simulink model "mcb_bldc_sixstep_f28069mLaunchPad_r2020a"  (R2020a)
settings: Solver=FixedStepDiscrete  StartTime=0.0  StopTime=2  RelTol=1e-3  EnableMultiTasking=on
InitFcn:
  | mcb_bldc_sixstep_f28069mLaunchPad_data;
undefined symbols (not defined in the file): bldc, Down, GPTRIP1SEL, GPTRIP2SEL, inverter, PI_params, PWM_frequency, target, Ts, Ts_motor, Ts_motor_simscape, Ts_simulink, Ts_speed, TZ1, TZ2, Up
libraries: nesl_utility x14, fl_lib x9, mcbcontrolslib x8, simulink x8, c2802xlib x7, mcbpositiondecoderlib x5, c2806xlib x5, c280xlib x5, ee_lib x5, svdschedulerlib x2
(part 1 of 3)
settings Model: SILPILModeSetting=veronly  SILPILSystemUnderTest=refmodels  ExtModeTrigDuration=8  OrderedModelArguments=off  Creator=The MathWorks, Inc.  LastModifiedBy=Tefilus
settings SolverCC: AutoInsertRateTranBlk=on
settings DataIOCC: LimitDataPoints=on  SaveFormat=Array  SaveOutput=off  SaveTime=off  ReturnWorkspaceOutputs=off
settings OptimizationCC: DefaultParameterBehavior=Inlined  DefaultUnderspecifiedDataType=single  OptimizeBlockIOStorage=off  BufferReuse=off  GlobalBufferReuse=off  ExpressionFolding=off  ExpressionDepthLimit=2147483647  LocalBlockOutputs=off  InitFltsAndDblsToZero=on  NoFixptDivByZeroProtection=on  EfficientFloat2IntCast=on  EfficientMapNaN2IntZero=off  LifeSpan=inf  MaxStackSize=1024  OptimizeDataStoreBuffers=off  BusAssignmentInplaceUpdate=off  DenormalBehavior=FlushToZero  EfficientTunableParamExpr=on
settings DebuggingCC: AlgebraicLoopMsg=error  ArtificialAlgebraicLoopMsg=error  CheckSSInitialOutputMsg=off  MergeDetectMultiDrivingBlocksExec=none  SolverPrmCheckMsg=warning  InheritedTsInSrcMsg=none  MultiTaskDSMMsg=none  MultiTaskCondExecSysMsg=none  TasksWithSamePriorityMsg=none  SigSpecEnsureSampleTimeMsg=none  ParameterPrecisionLossMsg=none  ParameterTunabilityLossMsg=error  FcnCallInpInsideContextMsg=warning  AllowSymbolicDim=off  StateNameClashWarn=warning  SFUnexpectedBacktrackingDiag=warning  SFNoUnconditionalDefaultTransitionDiag=warning  SFExecutionAtInitializationDiag=none  ArithmeticOperatorsInVariantConditions=warning
settings HardwareCC: ProdBitPerChar=16  ProdBitPerInt=16  ProdBitPerPointer=32  ProdBitPerSizeT=32  ProdBitPerPtrDiffT=32  ProdLargestAtomicInteger=Integer  ProdLargestAtomicFloat=None  ProdWordSize=16  ProdLongLongMode=on  ProdHWDeviceType=Texas Instruments->C2000  TargetBitPerChar=16  TargetBitPerInt=16  TargetLargestAtomicInteger=Integer  TargetLongLongMode=on  TargetIntDivRoundTo=Zero  TargetEndianess=LittleEndian  TargetWordSize=16  TargetHWDeviceType=Texas Instruments->C2000  ProdEqTarget=off
settings ModelReferenceCC: PropagateSignalLabelsOutOfModel=off
settings SFSimCC: SimUseLocalCustomCode=off  MATLABDynamicMemAlloc=off
settings RTWCC: SystemTargetFile=ert.tlc  HardwareBoard=TI Piccolo F28069M LaunchPad  TLCOptions=-aInlineSetEventsForThisBaseRateFcn=TLC_FALSE -aSuppressMultiTaskScheduler=TLC_FALSE -aRateBasedStepFcn=1  TemplateMakefile=ert_default_tmf  PostCodeGenCommand=; codertarget.postCodeGenHookCommand(h)  GenerateReport=on  RTWUseLocalCustomCode=off  Toolchain=Texas Instruments Code Composer Studio (C2000)  IncludeHyperlinkInReport=on  GenerateTraceInfo=on  GenerateTraceReport=on  GenerateTraceReportSl=on  GenerateTraceReportSf=on  GenerateTraceReportEml=on
settings CodeAppCC: IgnoreCustomStorageClasses=off  CustomSymbolStrType=$N$R$M  StateflowObjectComments=on  InternalIdentifier=Classic
settings ERTTargetCC: TargetFcnLib=ansi_tfl_tmw_new.mat  CodeReplacementLibrary=TI C28x  MultiwordLength=2048  ParMdlRefBuildCompliant=off  CompOptLevelCompliant=off  ConcurrentExecutionCompliant=off  CPPClassGenCompliant=off  ExtModeStaticAllocSize=2000  ExtModeMexFile=TIC2000ExternalModeOpen  ExtModeIntrfLevel=Level2 - Open  ConvertIfToSwitch=off  SuppressUnreachableDefaultCases=off  MemSecPackage=tic2000demospkg
settings ConfigComp: CovMetricSettings=dw  CovSaveCumulativeToWorkspaceVar=on  CovSaveSingleToWorkspaceVar=on  CovExternalEMLEnable=off  CovSFcnEnable=off

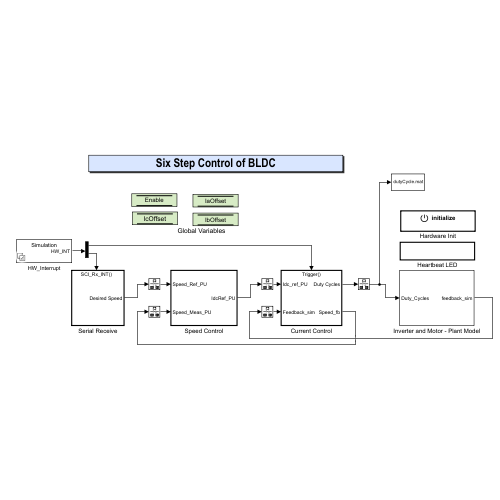
[thumbnail: Simulink's stored preview of the top-level diagram]
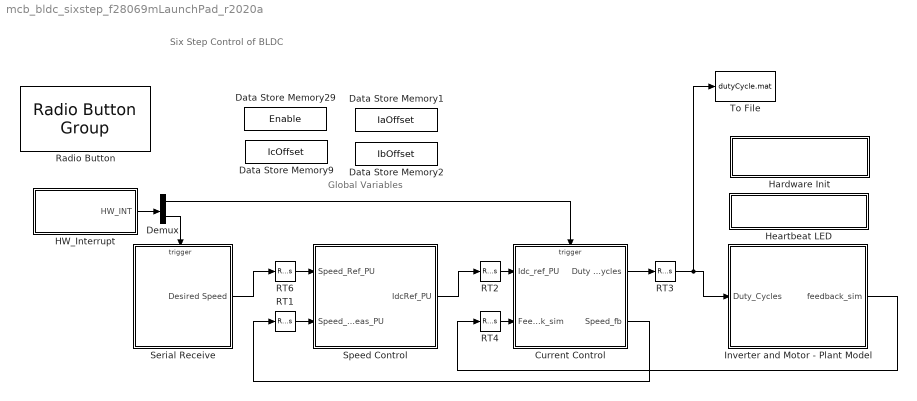
== system mcb_bldc_sixstep_f28069mLaunchPad_r2020a ==
  note: Six Step Control of BLDC
  note: Global Variables
  Current Control : Subsystem
      settings: RTWSystemCode=Nonreusable function
  Data Store Memory1 : DataStoreMemory  DataStoreName=IaOffset  InitialValue=inverter.CtSensAOffset  ShowAdditionalParam=off
  Data Store Memory2 : DataStoreMemory  DataStoreName=IbOffset  InitialValue=inverter.CtSensBOffset  ShowAdditionalParam=off
  Data Store Memory29 : DataStoreMemory  DataStoreName=Enable  ShowAdditionalParam=off  OutDataTypeStr=boolean
  Data Store Memory9 : DataStoreMemory  DataStoreName=IcOffset  InitialValue=inverter.CtSensBOffset  ShowAdditionalParam=off
  Demux : Demux  Outputs=2
  HW_Interrupt : Subsystem  Variant=on  VariantControlMode=Expression
  Hardware Init : Subsystem  TreatAsAtomicUnit=on
  Heartbeat LED : Subsystem  TreatAsAtomicUnit=on
  Inverter and Motor - Plant Model : Subsystem
  RT1 : RateTransition  Deterministic=off  OutPortSampleTime=Ts_speed
  RT{2..4,6} (4 alike) : RateTransition  Deterministic=off
  Radio Button : RadioButtonGroup  LabelPosition=Hide  SelectedLabel=Quadrature Encoder  ButtonGroupName=Speed_Feedback
      settings: Values={{'Quadrature Encoder', 'Hall'}, [0 1]}
  Serial Receive : Subsystem  SystemSampleTime=1e-3
  Speed Control : Subsystem  TreatAsAtomicUnit=on  SystemSampleTime=Ts_speed
  To File : ToFile  Filename=dutyCycle.mat  SaveFormat=Timeseries
  wires:
  RT3/1 -> To File/1, Inverter and Motor - Plant Model/1(Duty_Cycles)
  Inverter and Motor - Plant Model/1(feedback_sim) -> RT4/1
  Demux/1 -> Current Control/Trigger
  RT6/1 -> Speed Control/1(Speed_Ref_PU)
  RT1/1 -> Speed Control/2(Speed_Meas_PU)
  Speed Control/1(IdcRef_PU) -> RT2/1
  Demux/2 -> Serial Receive/Trigger
  Current Control/1(Duty Cycles) -> RT3/1
  HW_Interrupt/1(HW_INT) -> Demux/1
  Current Control/2(Speed_fb) -> RT1/1
  RT4/1 -> Current Control/2(Feedback_sim)
  Serial Receive/1(Desired Speed) -> RT6/1
  RT2/1 -> Current Control/1(Idc_ref_PU)

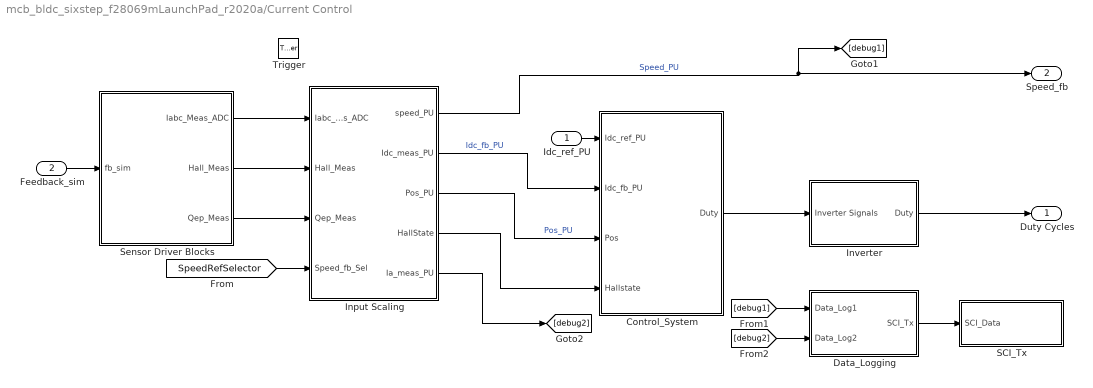
== system mcb_bldc_sixstep_f28069mLaunchPad_r2020a/Current Control ==
  Idc_ref_PU : Inport
  Feedback_sim : Inport  Port=2
  Trigger : TriggerPort  TriggerType=function-call  VariantControl=Variant  PortDimensions=1
  Control_System : Subsystem
  Data_Logging : Subsystem
  Input Scaling : Subsystem
  Inverter : Subsystem  Variant=on  VariantControlMode=Expression
  SCI_Tx : Subsystem  Variant=on  VariantControlMode=Expression
  Sensor Driver Blocks : Subsystem  Variant=on  VariantControlMode=Expression
  Duty Cycles : Outport  InitialOutput=0  VectorParamsAs1DForOutWhenUnconnected=off
  Speed_fb : Outport  Port=2  InitialOutput=0  VectorParamsAs1DForOutWhenUnconnected=off
  wires:
  [debug1] -> Data_Logging/1(Data_Log1)
  [debug2] -> Data_Logging/2(Data_Log2)
  Inverter/1(Duty) -> Duty Cycles/1
  Data_Logging/1(SCI_Tx) -> SCI_Tx/1(SCI_Data)
  [SpeedRefSelector] -> Input Scaling/4(Speed_fb_Sel)
  Sensor Driver Blocks/1(Iabc_Meas_ADC) -> Input Scaling/1(Iabc_meas_ADC)
  Feedback_sim/1 -> Sensor Driver Blocks/1(fb_sim)
  Idc_ref_PU/1 -> Control_System/1(Idc_ref_PU)
  Input Scaling/2(Idc_meas_PU) -> Control_System/2(Idc_fb_PU)  "Idc_fb_PU"
  Input Scaling/3(Pos_PU) -> Control_System/3(Pos)  "Pos_PU"
  Input Scaling/4(HallState) -> Control_System/4(Hallstate)
  Input Scaling/1(speed_PU) -> [debug1], Speed_fb/1  "Speed_PU"
  Input Scaling/5(Ia_meas_PU) -> [debug2]
  Sensor Driver Blocks/2(Hall_Meas) -> Input Scaling/2(Hall_Meas)
  Sensor Driver Blocks/3(Qep_Meas) -> Input Scaling/3(Qep_Meas)
  Control_System/1(Duty) -> Inverter/1(Inverter Signals)

== system mcb_bldc_sixstep_f28069mLaunchPad_r2020a/HW_Interrupt ==
  Code generation : Subsystem  VariantControl=(codegen)
  Simulation : Subsystem  VariantControl=(sim)
  HW_INT : Outport

== system mcb_bldc_sixstep_f28069mLaunchPad_r2020a/Hardware Init ==
  6PWM_Mode : Constant  Priority=1000  Value=0x3A16  OutDataTypeStr=uint16  SampleTime=-1
  ADC_Gain_Setting : Constant  Priority=1000  Value=inverter.SPI_Gain_Setting  OutDataTypeStr=uint16  SampleTime=-1
  Event Listener : EventListener  DisableCoverage=on  EventName=reset
  Mux : Mux  Inputs=2
  Variant Subsystem : Subsystem  Variant=on  VariantControlMode=Expression
  wires:
  6PWM_Mode/1 -> Mux/1
  ADC_Gain_Setting/1 -> Mux/2
  Mux/1 -> Variant Subsystem/1(In1)

== system mcb_bldc_sixstep_f28069mLaunchPad_r2020a/Heartbeat LED ==
  note: Heartbeat LED 1HZ
  Heartbeat LED : Subsystem  Variant=on  VariantControlMode=Expression
  RED_LED : Constant  OutDataTypeStr=uint16  SampleTime=0.5
  wires:
  RED_LED/1 -> Heartbeat LED/1(In1)

== system mcb_bldc_sixstep_f28069mLaunchPad_r2020a/Inverter and Motor - Plant Model ==
  Duty_Cycles : Inport
  Codegeneration : Subsystem
  Simulation : Subsystem
  Variant Sink : VariantSink  VariantControlMode=Expression
  Variant Source : VariantSource  VariantControlMode=Expression
  feedback_sim : Outport  VectorParamsAs1DForOutWhenUnconnected=off
  wires:
  Codegeneration/1(fb_codegen) -> Variant Source/1
  Variant Sink/1 -> Codegeneration/1(Duty_Cycles)
  Variant Source/1 -> feedback_sim/1
  Duty_Cycles/1 -> Variant Sink/1
  Variant Sink/2 -> Simulation/1(Duty_Cycles)
  Simulation/1(fb_sim) -> Variant Source/2

== system mcb_bldc_sixstep_f28069mLaunchPad_r2020a/Serial Receive ==
  SCI_Rx_INT : TriggerPort  TriggerType=function-call  VariantControl=Variant
  Data Store Write : DataStoreWrite  DataStoreName=Enable
  Data Type Conversion1 : DataTypeConversion  OutDataTypeStr=dataType  RndMeth=Simplest
  Data Type Conversion3 : DataTypeConversion  OutDataTypeStr=boolean  RndMeth=Simplest
  Data_Conditioning : Subsystem
  Demux : Demux  Outputs=2
  SCI_Rx : Subsystem  Variant=on  VariantControlMode=Expression
  Desired Speed : Outport  VectorParamsAs1DForOutWhenUnconnected=off
  wires:
  SCI_Rx/1(Data) -> Data_Conditioning/1(In1)
  Data Type Conversion1/1 -> Desired Speed/1
  Demux/2 -> Data Type Conversion3/1
  Data_Conditioning/1(Out1) -> Demux/1
  Demux/1 -> Data Type Conversion1/1
  Data Type Conversion3/1 -> Data Store Write/1

== system mcb_bldc_sixstep_f28069mLaunchPad_r2020a/Speed Control ==
  Speed_Ref_PU : Inport
  Speed_Meas_PU : Inport  Port=2
  PI_Controller_Speed : Subsystem
  Scope : Scope  NumInputPorts=2
  Speed_Ref_Selector : Subsystem
  IdcRef_PU : Outport  VectorParamsAs1DForOutWhenUnconnected=off
  wires:
  PI_Controller_Speed/1(Idc_ref) -> IdcRef_PU/1
  Speed_Meas_PU/1 -> Scope/2, PI_Controller_Speed/2(N_fb), Speed_Ref_Selector/2(Speed_Ref_Open)  "Speed_fb"
  Speed_Ref_PU/1 -> Speed_Ref_Selector/1(Speed_Ref_In)  "SpeedRef"
  Speed_Ref_Selector/1(Speed_Ref_PU) -> Scope/1, PI_Controller_Speed/1(N_ref)  "Speed_Ref"

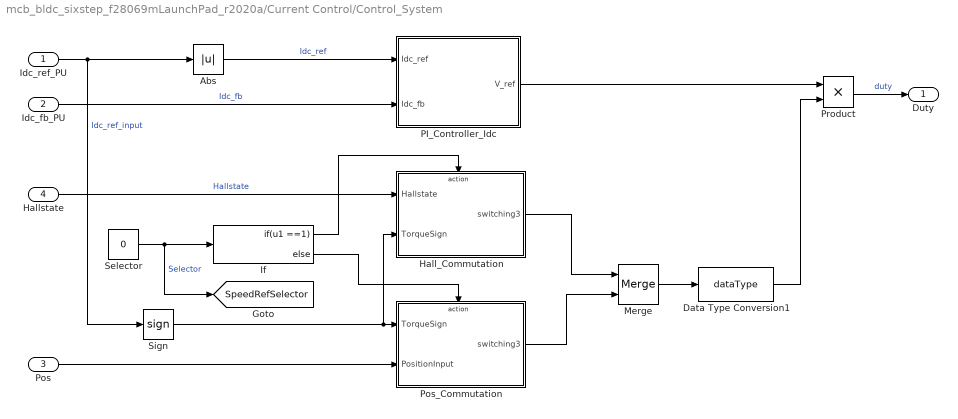
== system mcb_bldc_sixstep_f28069mLaunchPad_r2020a/Current Control/Control_System ==
  Idc_ref_PU : Inport
  Idc_fb_PU : Inport  Port=2
  Pos : Inport  Port=3
  Hallstate : Inport  Port=4
  Abs : Abs
  Data Type Conversion1 : DataTypeConversion  OutDataTypeStr=dataType  RndMeth=Simplest
  Hall_Commutation : Subsystem
  If : If  IfExpression=u1 ==1
  Merge : Merge
  PI_Controller_Idc : Subsystem
  Pos_Commutation : Subsystem
  Product : Product  RndMeth=Simplest  OutDataTypeStr=Inherit: Same as first input
  Selector : Constant  Value=0  OutDataTypeStr=uint16  SampleTime=-1
  Sign : Signum
  Duty : Outport  VectorParamsAs1DForOutWhenUnconnected=off
  tag scope: SpeedRefSelector=global
  wires:
  Hallstate/1 -> Hall_Commutation/1(Hallstate)  "Hallstate"
  Pos/1 -> Pos_Commutation/2(PositionInput)
  If/1 -> Hall_Commutation/Action
  If/2 -> Pos_Commutation/Action
  Pos_Commutation/1(switching3) -> Merge/2
  Hall_Commutation/1(switching3) -> Merge/1
  Merge/1 -> Data Type Conversion1/1
  Idc_fb_PU/1 -> PI_Controller_Idc/2(Idc_fb)  "Idc_fb"
  Abs/1 -> PI_Controller_Idc/1(Idc_ref)  "Idc_ref"
  PI_Controller_Idc/1(V_ref) -> Product/1
  Idc_ref_PU/1 -> Sign/1, Abs/1  "Idc_ref_input"
  Product/1 -> Duty/1  "duty"
  Selector/1 -> [SpeedRefSelector], If/1  "Selector"
  Sign/1 -> Hall_Commutation/2(TorqueSign), Pos_Commutation/1(TorqueSign)
  Data Type Conversion1/1 -> Product/2

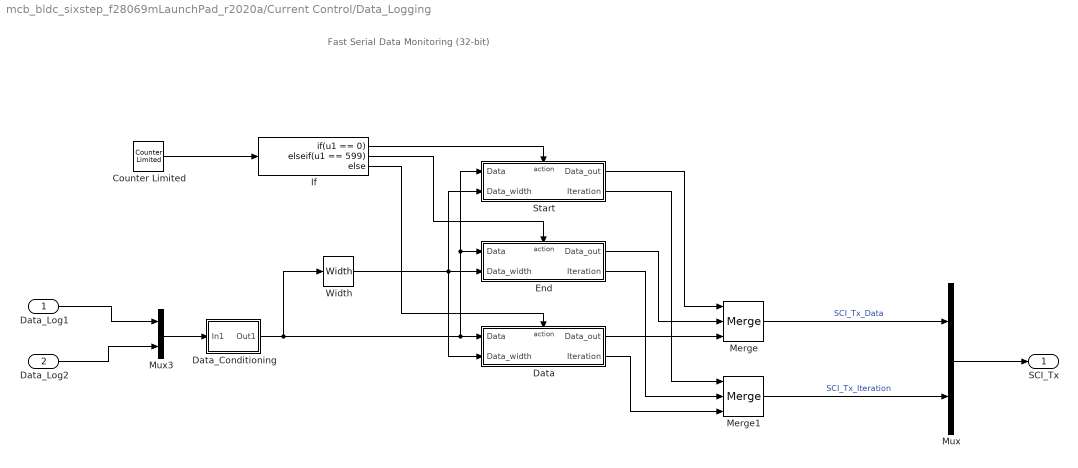
== system mcb_bldc_sixstep_f28069mLaunchPad_r2020a/Current Control/Data_Logging ==
  note: Fast Serial Data Monitoring (32-bit)
  Data_Log1 : Inport
  Data_Log2 : Inport  Port=2
  Counter Limited : simulink/Sources/Counter Limited  uplimit=599  tsamp=-1
  Data : Subsystem  TreatAsAtomicUnit=on
  Data_Conditioning : Subsystem
  End : Subsystem  TreatAsAtomicUnit=on
  If : If  IfExpression=u1 == 0  ElseIfExpressions=u1 == 599
  Merge : Merge  Inputs=3
  Merge1 : Merge  Inputs=3
  Mux : Mux  Inputs=2
  Mux3 : Mux  Inputs=2
  Start : Subsystem  TreatAsAtomicUnit=on
  Width : Width  OutDataTypeMode=All ports same datatype  DataType=uint16
  SCI_Tx : Outport
  wires:
  If/3 -> Data/Action
  Data/1(Data_out) -> Merge/3
  Width/1 -> Data/2(Data_width), Start/2(Data_width), End/2(Data_width)
  Merge/1 -> Mux/1  "SCI_Tx_Data"
  Counter Limited/1 -> If/1
  Start/2(Iteration) -> Merge1/1
  Start/1(Data_out) -> Merge/1
  If/2 -> End/Action
  Merge1/1 -> Mux/2  "SCI_Tx_Iteration"
  If/1 -> Start/Action
  End/1(Data_out) -> Merge/2
  End/2(Iteration) -> Merge1/2
  Data/2(Iteration) -> Merge1/3
  Data_Log1/1 -> Mux3/1
  Data_Conditioning/1(Out1) -> Width/1, Start/1(Data), End/1(Data), Data/1(Data)
  Mux/1 -> SCI_Tx/1
  Mux3/1 -> Data_Conditioning/1(In1)
  Data_Log2/1 -> Mux3/2

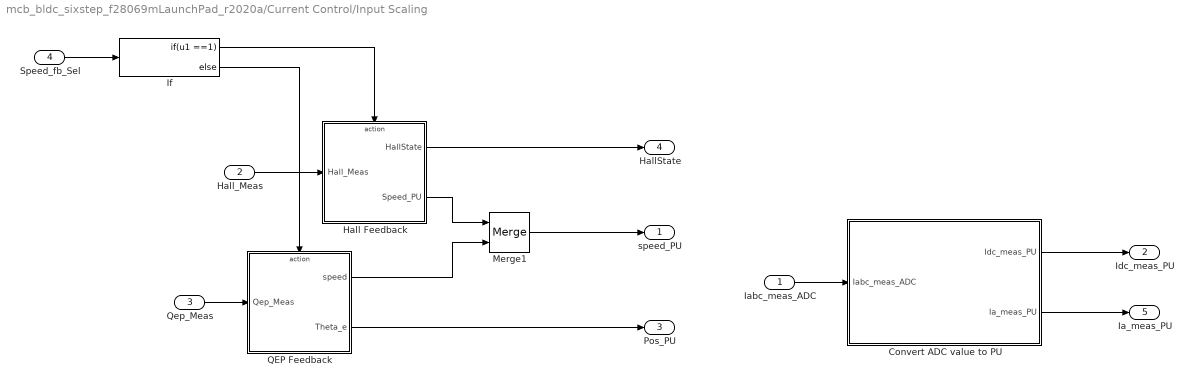
== system mcb_bldc_sixstep_f28069mLaunchPad_r2020a/Current Control/Input Scaling ==
  Iabc_meas_ADC : Inport
  Hall_Meas : Inport  Port=2
  Qep_Meas : Inport  Port=3
  Speed_fb_Sel : Inport  Port=4
  Convert ADC value to PU : Subsystem
  Hall Feedback : Subsystem  TreatAsAtomicUnit=on
  If : If  IfExpression=u1 ==1
  Merge1 : Merge
  QEP Feedback : Subsystem  TreatAsAtomicUnit=on
  speed_PU : Outport  InitialOutput=0  VectorParamsAs1DForOutWhenUnconnected=off
  Idc_meas_PU : Outport  Port=2  VectorParamsAs1DForOutWhenUnconnected=off
  Pos_PU : Outport  Port=3  InitialOutput=0  VectorParamsAs1DForOutWhenUnconnected=off
  HallState : Outport  Port=4  InitialOutput=0  VectorParamsAs1DForOutWhenUnconnected=off
  Ia_meas_PU : Outport  Port=5  VectorParamsAs1DForOutWhenUnconnected=off
  wires:
  If/2 -> QEP Feedback/Action
  Convert ADC value to PU/2(Ia_meas_PU) -> Ia_meas_PU/1
  Convert ADC value to PU/1(Idc_meas_PU) -> Idc_meas_PU/1
  QEP Feedback/1(speed) -> Merge1/2
  Hall Feedback/2(Speed_PU) -> Merge1/1
  Iabc_meas_ADC/1 -> Convert ADC value to PU/1(Iabc_meas_ADC)
  QEP Feedback/2(Theta_e) -> Pos_PU/1
  Merge1/1 -> speed_PU/1
  Speed_fb_Sel/1 -> If/1
  Hall_Meas/1 -> Hall Feedback/1(Hall_Meas)
  Qep_Meas/1 -> QEP Feedback/1(Qep_Meas)
  If/1 -> Hall Feedback/Action
  Hall Feedback/1(HallState) -> HallState/1

== system mcb_bldc_sixstep_f28069mLaunchPad_r2020a/Current Control/Inverter ==
  Inverter Signals : Inport
  " Code Generation" : Subsystem  VariantControl=(codegen)
  Simulation : Subsystem  VariantControl=(sim)
  Duty : Outport  VectorParamsAs1DForOutWhenUnconnected=off

== system mcb_bldc_sixstep_f28069mLaunchPad_r2020a/Current Control/SCI_Tx ==
  SCI_Data : Inport
  " Code Generation" : Subsystem  VariantControl=(codegen)
  Simulation : Subsystem  VariantControl=(sim)

== system mcb_bldc_sixstep_f28069mLaunchPad_r2020a/Current Control/Sensor Driver Blocks ==
  fb_sim : Inport
  Sensor Driver Blocks (codegen) : Subsystem  VariantControl=(codegen)
  Sensor Driver Blocks (sim) : Subsystem  VariantControl=(sim)
  Iabc_Meas_ADC : Outport
  Hall_Meas : Outport  Port=2
  Qep_Meas : Outport  Port=3

== system mcb_bldc_sixstep_f28069mLaunchPad_r2020a/HW_Interrupt/Code generation ==
  HWI_ADCINT1 : svdschedulerlib/Hardware Interrupt v2  ISRGroup=ADC - Analog to Digital Converter  ISRName=ADCA1_INT  ISRNumber=32  NumEventsToServe=1  EventsList={'on','EOC event','1';'off','Overflow event','2';'off','Custom event','3'}  SelectedEvents={'event1'}  TaskPriority=30  DisablePreemption=off  ClearInterruptFlagsAtEndOfEvent=on  InterruptDefinitionFile=$(TARGET_ROOT)/registry/interrupts/F2837xS_interrupts.xml  HardwareBoard=F2837x  EnableSimPort=off
  HWI_SCIRXINTA : svdschedulerlib/Hardware Interrupt v2  ISRGroup=ADC - Analog to Digital Converter  ISRName=ADCA1_INT  ISRNumber=32  NumEventsToServe=1  EventsList={'on','EOC event','1';'off','Overflow event','2';'off','Custom event','3'}  SelectedEvents={'event1'}  TaskPriority=50  DisablePreemption=on  ClearInterruptFlagsAtEndOfEvent=on  InterruptDefinitionFile=$(TARGET_ROOT)/registry/interrupts/F2837xS_interrupts.xml  HardwareBoard=F2837x  EnableSimPort=off
  Mux : Mux  Inputs=2
  HW_INT : Outport
  wires:
  HWI_SCIRXINTA/1 -> Mux/2
  HWI_ADCINT1/1 -> Mux/1
  Mux/1 -> HW_INT/1

== system mcb_bldc_sixstep_f28069mLaunchPad_r2020a/HW_Interrupt/Simulation ==
  ADCINT1 : simulink/Ports & Subsystems/Function-Call Generator  sample_time=Ts  numberOfIterations=1  DisallowWideOutput=off
  Mux : Mux  Inputs=2
  SCI_Rx_INT : simulink/Ports & Subsystems/Function-Call Generator  sample_time=0.1  numberOfIterations=1  DisallowWideOutput=off
  HW_INT : Outport
  wires:
  SCI_Rx_INT/1 -> Mux/2
  ADCINT1/1 -> Mux/1
  Mux/1 -> HW_INT/1

== system mcb_bldc_sixstep_f28069mLaunchPad_r2020a/Hardware Init/Variant Subsystem ==
  In1 : Inport
  Code Generation : Subsystem  VariantControl=(codegen)
  Simulation : Subsystem  VariantControl=(sim)

== system mcb_bldc_sixstep_f28069mLaunchPad_r2020a/Heartbeat LED/Heartbeat LED ==
  In1 : Inport
  Code generation : Subsystem  VariantControl=(codegen)
  Simulation : Subsystem  VariantControl=(sim)

== system mcb_bldc_sixstep_f28069mLaunchPad_r2020a/Inverter and Motor - Plant Model/Codegeneration ==
  Duty_Cycles : Inport
  Bus Creator : BusCreator  Inputs=3
  Ground : Ground
  Terminator : Terminator
  fb_codegen : Outport  VectorParamsAs1DForOutWhenUnconnected=off
  wires:
  Duty_Cycles/1 -> Terminator/1
  Bus Creator/1 -> fb_codegen/1
  Ground/1 -> Bus Creator/3, Bus Creator/2, Bus Creator/1

== system mcb_bldc_sixstep_f28069mLaunchPad_r2020a/Inverter and Motor - Plant Model/Simulation ==
  Duty_Cycles : Inport
  Bus Creator : BusCreator  Inputs=3
  Inverter and Motor : Subsystem  VariantControl=get_param([bdroot '/Plant'],'Value')=='0'
  Load_Profile (Torque) : Subsystem
  RT1 : RateTransition  Deterministic=off  OutPortSampleTime=Ts_simulink
  RT2 : RateTransition  Deterministic=off  OutPortSampleTime=Ts_simulink
  RT3 : RateTransition  Deterministic=off  OutPortSampleTime=Ts_simulink
  Sensor_Measurements : Subsystem
  fb_sim : Outport
  wires:
  RT2/1 -> Sensor_Measurements/3(Hall)
  Sensor_Measurements/2(Pos_mech) -> Bus Creator/2  "Pos_fb"
  RT1/1 -> Sensor_Measurements/2(Pos)
  Bus Creator/1 -> fb_sim/1
  Sensor_Measurements/1(Iabc meas ADC) -> Bus Creator/1  "Iabc_fb"
  Sensor_Measurements/3(HallState) -> Bus Creator/3  "Hall_fb"
  Duty_Cycles/1 -> Inverter and Motor/1(Duty_Cycles)
  Load_Profile (Torque)/1(Load_Trq) -> Inverter and Motor/2(Load)
  Inverter and Motor/1(Iabc) -> RT3/1
  Inverter and Motor/2(Theta) -> RT1/1
  Inverter and Motor/3(Hall) -> RT2/1
  RT3/1 -> Sensor_Measurements/1(Iabc meas)

== system mcb_bldc_sixstep_f28069mLaunchPad_r2020a/Serial Receive/Data_Conditioning ==
  In1 : Inport
  Data Type Conversion1 : DataTypeConversion  OutDataTypeStr=single  RndMeth=Simplest
  Data Type Conversion2 : DataTypeConversion  OutDataTypeStr=fixdt(1,16,12)  ConvertRealWorld=Stored Integer (SI)  RndMeth=Simplest
  Out1 : Outport  VectorParamsAs1DForOutWhenUnconnected=off
  wires:
  Data Type Conversion1/1 -> Out1/1
  In1/1 -> Data Type Conversion2/1
  Data Type Conversion2/1 -> Data Type Conversion1/1

== system mcb_bldc_sixstep_f28069mLaunchPad_r2020a/Serial Receive/SCI_Rx ==
  Code Generation : Subsystem  VariantControl=(codegen)
  Simulation : Subsystem  VariantControl=(sim)
  Data : Outport

== system mcb_bldc_sixstep_f28069mLaunchPad_r2020a/Speed Control/PI_Controller_Speed ==
  N_ref : Inport
  N_fb : Inport  Port=2
  Data Store Read2 : DataStoreRead  DataStoreName=Enable
  Discrete PI Controller with anti-windup & reset : mcbcontrolslib/Discrete PI Controller  with anti-windup & reset  Controller=PI  UpperSaturationLimit=1  LowerSaturationLimit=-1  IntegratorRTWStateStorageClass=Auto  FilterRTWStateStorageClass=Auto  ParallelPVariant=ExternalParameters  IdealPVariant=Disabled  IVariant=ExternalParameters  DVariant=Disabled  IntegratorVariant=Discrete  SatVariant=Enabled  AWVariant=DiscClampingParallel  PCopyVariant=Disabled  TRVariant=Disabled  FdbkBlocksVariant=Forward  IdealPFdbkVariant=Disabled  SatFdbkVariant=Disabled  DerivativeFilterVariant=Disabled  NVariant=Disabled  NCopyVariant=Disabled_SignalSpec  FilterICVariant=Disabled  IntegratorICVariant=ExternalICs  ExternalResetVariant=ExternalReset  TRSumVariant=Passthrough  SumFdbkVariant=Disabled  SumVariant=Sum_PI  TsampFilterVariant=InternalTs  TsampNgainVariant=Passthrough  TsampIntegralVariant=Disabled_SignalSpec
  Ki1 : Constant  Value=PI_params.Ki_speed*Ts_speed  OutDataTypeStr=dataType  SampleTime=-1
  Ki2 : Constant  Value=0  OutDataTypeStr=dataType  SampleTime=-1
  Kp1 : Constant  Value=PI_params.Kp_speed  OutDataTypeStr=dataType  SampleTime=-1
  Logical Operator : Logic  Operator=NOT  IconShape=distinctive  AllPortsSameDT=off  OutDataTypeStr=boolean
  Sum : Sum  Inputs=|+-  RndMeth=Round
  Zero_Cancellation : mcbcontrolslib/IIR Filter  VariantControl=Low Pass Filter  VariantSelect=Low-pass  Filter_constant=0.01*(Ts_speed/Ts)  advancedSettings=off  Ts=50e-6  cutOff_freq=1
  Idc_ref : Outport  VectorParamsAs1DForOutWhenUnconnected=off
  wires:
  Discrete PI Controller with anti-windup & reset/1 -> Idc_ref/1
  Ki1/1 -> Discrete PI Controller with anti-windup & reset/3
  Kp1/1 -> Discrete PI Controller with anti-windup & reset/2
  N_fb/1 -> Sum/2
  N_ref/1 -> Zero_Cancellation/1
  Logical Operator/1 -> Discrete PI Controller with anti-windup & reset/4
  Ki2/1 -> Discrete PI Controller with anti-windup & reset/5
  Sum/1 -> Discrete PI Controller with anti-windup & reset/1
  Data Store Read2/1 -> Logical Operator/1
  Zero_Cancellation/1 -> Sum/1

== system mcb_bldc_sixstep_f28069mLaunchPad_r2020a/Speed Control/Speed_Ref_Selector ==
  Speed_Ref_In : Inport
  Speed_Ref_Open : Inport  Port=2
  Data Store Read1 : DataStoreRead  DataStoreName=Enable
  Switch : Switch  Criteria=u2 > Threshold  Threshold=0.5
  Speed_Ref_PU : Outport
  wires:
  Switch/1 -> Speed_Ref_PU/1
  Data Store Read1/1 -> Switch/2
  Speed_Ref_Open/1 -> Switch/3
  Speed_Ref_In/1 -> Switch/1

== system mcb_bldc_sixstep_f28069mLaunchPad_r2020a/Current Control/Control_System/Hall_Commutation ==
  Hallstate : Inport
  TorqueSign : Inport  Port=2
  Action Port : ActionPort  ActionPortLabel=if(u1 ==1)
  Six Step Commutation : mcbcontrolslib/Six Step Commutation  InputType=Hall  PositionUnit=Per unit  CommutationMode=120 deg  SequencePos=bldc.HallSequence  EnableCustomSwitching=on  CommutationSeqPos=hallCommutation  CommutationSeqNeg="[0  1  1  0  0  0;0  1  0  0  1  0;0  0  0  1  1  0;1  0  0  1  0  0;1  0  0  0  0  1;0  0  1  0  0  1;]"
  switching3 : Outport
  wires:
  Hallstate/1 -> Six Step Commutation/1
  Six Step Commutation/1 -> switching3/1  "switching"
  TorqueSign/1 -> Six Step Commutation/2

== system mcb_bldc_sixstep_f28069mLaunchPad_r2020a/Current Control/Control_System/PI_Controller_Idc ==
  Idc_ref : Inport
  Idc_fb : Inport  Port=2
  Data Store Read1 : DataStoreRead  DataStoreName=Enable
  Discrete PI Controller with anti-windup & reset : mcbcontrolslib/Discrete PI Controller  with anti-windup & reset  Controller=PI  UpperSaturationLimit=1  LowerSaturationLimit=0  IntegratorRTWStateStorageClass=Auto  FilterRTWStateStorageClass=Auto  ParallelPVariant=ExternalParameters  IdealPVariant=Disabled  IVariant=ExternalParameters  DVariant=Disabled  IntegratorVariant=Discrete  SatVariant=Enabled  AWVariant=DiscClampingParallel  PCopyVariant=Disabled  TRVariant=Disabled  FdbkBlocksVariant=Forward  IdealPFdbkVariant=Disabled  SatFdbkVariant=Disabled  DerivativeFilterVariant=Disabled  NVariant=Disabled  NCopyVariant=Disabled_SignalSpec  FilterICVariant=Disabled  IntegratorICVariant=ExternalICs  ExternalResetVariant=ExternalReset  TRSumVariant=Passthrough  SumFdbkVariant=Disabled  SumVariant=Sum_PI  TsampFilterVariant=InternalTs  TsampNgainVariant=Passthrough  TsampIntegralVariant=Disabled_SignalSpec
  Ki : Constant  Value=PI_params.Ki_i*Ts  OutDataTypeStr=dataType  SampleTime=-1
  Kp : Constant  Value=PI_params.Kp_i  OutDataTypeStr=dataType  SampleTime=-1
  Kp1 : Constant  Value=0  OutDataTypeStr=dataType  SampleTime=-1
  Logical Operator : Logic  Operator=NOT  IconShape=distinctive  AllPortsSameDT=off  OutDataTypeStr=boolean
  Sum : Sum  Inputs=|+-  OutDataTypeStr=Inherit: Same as first input
  V_ref : Outport  VectorParamsAs1DForOutWhenUnconnected=off
  wires:
  Discrete PI Controller with anti-windup & reset/1 -> V_ref/1
  Data Store Read1/1 -> Logical Operator/1
  Idc_fb/1 -> Sum/2
  Idc_ref/1 -> Sum/1
  Sum/1 -> Discrete PI Controller with anti-windup & reset/1
  Logical Operator/1 -> Discrete PI Controller with anti-windup & reset/4
  Kp1/1 -> Discrete PI Controller with anti-windup & reset/5
  Kp/1 -> Discrete PI Controller with anti-windup & reset/2
  Ki/1 -> Discrete PI Controller with anti-windup & reset/3

== system mcb_bldc_sixstep_f28069mLaunchPad_r2020a/Current Control/Control_System/Pos_Commutation ==
  TorqueSign : Inport
  PositionInput : Inport  Port=2
  Action Port : ActionPort  ActionPortLabel=else
  Six Step Commutation : mcbcontrolslib/Six Step Commutation  InputType=Position  PositionUnit=Per unit  CommutationMode=120 deg  SequencePos=[5,4,6,2,3,1]  EnableCustomSwitching=off  CommutationSeqPos=[1 0 0 1 0 0;1 0 0 0 0 1; 0 0 1 0 0 1;0 1 1 0 0 0;0 1 0 0 1 0;0 0 0 1 1 0]  CommutationSeqNeg="[0  1  1  0  0  0;0  1  0  0  1  0;0  0  0  1  1  0;1  0  0  1  0  0;1  0  0  0  0  1;0  0  1  0  0  1;]"
  switching3 : Outport
  wires:
  PositionInput/1 -> Six Step Commutation/1
  TorqueSign/1 -> Six Step Commutation/2
  Six Step Commutation/1 -> switching3/1  "switching"

== system mcb_bldc_sixstep_f28069mLaunchPad_r2020a/Current Control/Data_Logging/Data ==
  Data : Inport
  Data_width : Inport  Port=2
  Action Port : ActionPort  ActionPortLabel=else
  Mux : Mux  Inputs=2
  Start : Constant  Value=hex2dec('0000')  OutDataTypeStr=uint16
  Data_out : Outport  VectorParamsAs1DForOutWhenUnconnected=off
  Iteration : Outport  Port=2  VectorParamsAs1DForOutWhenUnconnected=off
  wires:
  Start/1 -> Mux/2
  Mux/1 -> Data_out/1
  Data/1 -> Mux/1
  Data_width/1 -> Iteration/1

== system mcb_bldc_sixstep_f28069mLaunchPad_r2020a/Current Control/Data_Logging/Data_Conditioning ==
  In1 : Inport
  Data Type Conversion : DataTypeConversion  OutDataTypeStr=fixdt(1,16,12)  RndMeth=Simplest
  Data Type Conversion3 : DataTypeConversion  OutDataTypeStr=uint16  ConvertRealWorld=Stored Integer (SI)
  Out1 : Outport  VectorParamsAs1DForOutWhenUnconnected=off
  wires:
  In1/1 -> Data Type Conversion/1
  Data Type Conversion3/1 -> Out1/1
  Data Type Conversion/1 -> Data Type Conversion3/1

== system mcb_bldc_sixstep_f28069mLaunchPad_r2020a/Current Control/Data_Logging/End ==
  Data : Inport
  Data_width : Inport  Port=2
  Action Port : ActionPort  ActionPortLabel=elseif(u1 == 599)
  Bias : Bias  Bias=1
  Mux : Mux  Inputs=2
  Start : Constant  Value=hex2dec('4545')  OutDataTypeStr=uint16
  Data_out : Outport  VectorParamsAs1DForOutWhenUnconnected=off
  Iteration : Outport  Port=2  VectorParamsAs1DForOutWhenUnconnected=off
  wires:
  Mux/1 -> Data_out/1
  Data_width/1 -> Bias/1
  Start/1 -> Mux/2
  Bias/1 -> Iteration/1
  Data/1 -> Mux/1

== system mcb_bldc_sixstep_f28069mLaunchPad_r2020a/Current Control/Data_Logging/Start ==
  Data : Inport
  Data_width : Inport  Port=2
  Action Port : ActionPort  ActionPortLabel=if(u1 == 0)
  Bias : Bias  Bias=1
  End : Constant  Value=hex2dec('5353')  OutDataTypeStr=uint16
  Mux : Mux  Inputs=2
  Data_out : Outport  VectorParamsAs1DForOutWhenUnconnected=off
  Iteration : Outport  Port=2  VectorParamsAs1DForOutWhenUnconnected=off
  wires:
  End/1 -> Mux/1
  Mux/1 -> Data_out/1
  Data_width/1 -> Bias/1
  Bias/1 -> Iteration/1
  Data/1 -> Mux/2

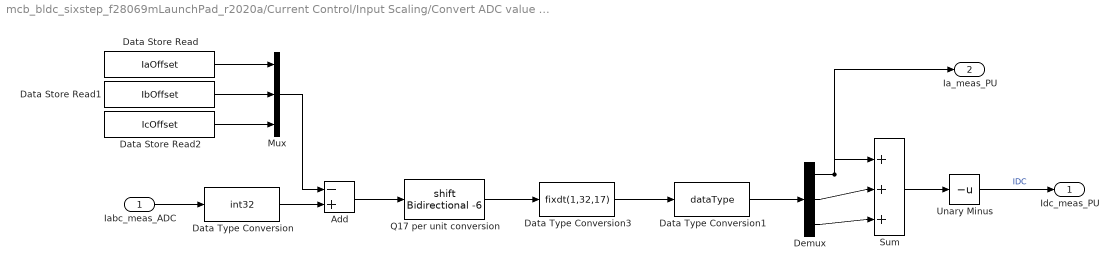
== system mcb_bldc_sixstep_f28069mLaunchPad_r2020a/Current Control/Input Scaling/Convert ADC value to PU ==
  Iabc_meas_ADC : Inport
  Add : Sum  Inputs=-+
  Data Store Read : DataStoreRead  DataStoreName=IaOffset
  Data Store Read1 : DataStoreRead  DataStoreName=IbOffset
  Data Store Read2 : DataStoreRead  DataStoreName=IcOffset
  Data Type Conversion : DataTypeConversion  OutDataTypeStr=int32  ConvertRealWorld=Stored Integer (SI)
  Data Type Conversion1 : DataTypeConversion  OutDataTypeStr=dataType
  Data Type Conversion3 : DataTypeConversion  OutDataTypeStr=fixdt(1,32,17)  ConvertRealWorld=Stored Integer (SI)  RndMeth=Simplest
  Demux : Demux  Outputs=3
  Mux : Mux  Inputs=3
  Q17 per unit conversion : ArithShift  BitShiftNumber=-6
  Sum : Sum  Inputs=|+++
  Unary Minus : UnaryMinus
  Idc_meas_PU : Outport
  Ia_meas_PU : Outport  Port=2  VectorParamsAs1DForOutWhenUnconnected=off
  wires:
  Data Type Conversion3/1 -> Data Type Conversion1/1
  Q17 per unit conversion/1 -> Data Type Conversion3/1
  Unary Minus/1 -> Idc_meas_PU/1  "IDC"
  Demux/2 -> Sum/2
  Demux/1 -> Sum/1, Ia_meas_PU/1
  Sum/1 -> Unary Minus/1
  Demux/3 -> Sum/3
  Data Type Conversion1/1 -> Demux/1
  Data Store Read2/1 -> Mux/3
  Data Store Read1/1 -> Mux/2
  Data Store Read/1 -> Mux/1
  Iabc_meas_ADC/1 -> Data Type Conversion/1
  Data Type Conversion/1 -> Add/2
  Mux/1 -> Add/1
  Add/1 -> Q17 per unit conversion/1

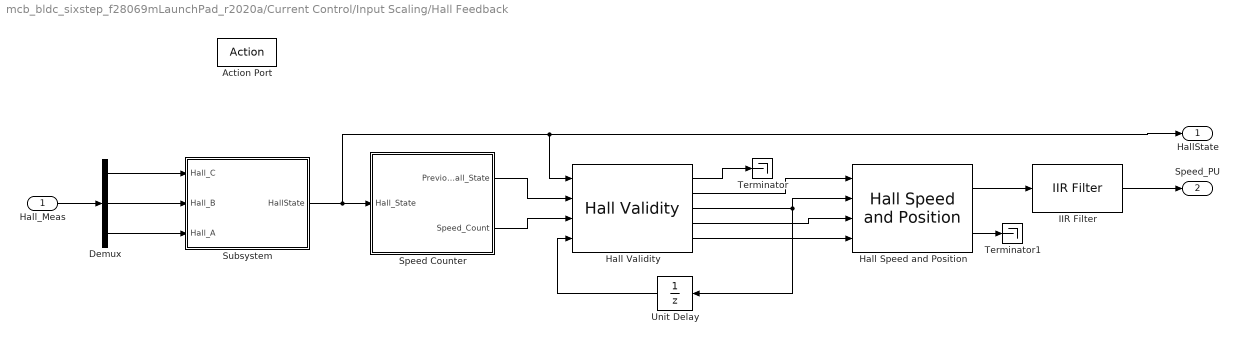
== system mcb_bldc_sixstep_f28069mLaunchPad_r2020a/Current Control/Input Scaling/Hall Feedback ==
  Hall_Meas : Inport
  Action Port : ActionPort  ActionPortLabel=if(u1 ==1)
  Demux : Demux  Outputs=3
  Hall Speed and Position : mcbpositiondecoderlib/Hall Speed and Position  blkExecutionType=Speed  CounterSize=32 bits  ClkFreq=1/Ts  BlkSampleTime=Ts  PolePairs=bldc.p  MinSpeed=20  HallInterruptConfig=Every 60 Degrees  SpeedUnit=Per unit  PerUnitSpeed=PU_System.N_base  SpeedDataType=dataType  hallSequence=ABC  Sequence=[5,4,6,2,3,1]  EnableSecondOrder=1st Order  PositionUnit=Radians  PositionDataType=single
  Hall Validity : mcbpositiondecoderlib/Hall Validity  hallSequence=Custom sequence  sequence=bldc.HallSequence  CounterSize=32 bits
  IIR Filter : mcbcontrolslib/IIR Filter  VariantControl=Low Pass Filter  VariantSelect=Low-pass  Filter_constant=0.01  advancedSettings=off  Ts=50e-6  cutOff_freq=32.1525
  Speed Counter : Subsystem
  Subsystem : Subsystem
  Terminator : Terminator
  Terminator1 : Terminator
  Unit Delay : UnitDelay  InitialCondition=1  SampleTime=-1  HasFrameUpgradeWarning=on
  HallState : Outport  InitialOutput=0  VectorParamsAs1DForOutWhenUnconnected=off
  Speed_PU : Outport  Port=2  InitialOutput=0  VectorParamsAs1DForOutWhenUnconnected=off
  wires:
  Hall Speed and Position/1 -> IIR Filter/1
  Hall Speed and Position/2 -> Terminator1/1
  Hall Validity/2 -> Hall Speed and Position/1
  Hall Validity/3 -> Hall Speed and Position/2, Unit Delay/1
  Hall Validity/4 -> Hall Speed and Position/3
  Hall Validity/5 -> Hall Speed and Position/4
  Speed Counter/2(Speed_Count) -> Hall Validity/3
  Speed Counter/1(Previous_Hall_State) -> Hall Validity/2
  Subsystem/1(HallState) -> HallState/1, Hall Validity/1, Speed Counter/1(Hall_State)
  Unit Delay/1 -> Hall Validity/4
  Hall Validity/1 -> Terminator/1
  IIR Filter/1 -> Speed_PU/1
  Demux/1 -> Subsystem/1(Hall_C)
  Demux/2 -> Subsystem/2(Hall_B)
  Demux/3 -> Subsystem/3(Hall_A)
  Hall_Meas/1 -> Demux/1

== system mcb_bldc_sixstep_f28069mLaunchPad_r2020a/Current Control/Input Scaling/QEP Feedback ==
  Qep_Meas : Inport
  Action Port : ActionPort  ActionPortLabel=else
  " Calculate Position and Speed" : Subsystem
  Demux : Demux  Outputs=2
  IndexOffset : Constant  Value=bldc.PositionOffset  OutDataTypeStr=dataType  SampleTime=-1
  speed : Outport
  Theta_e : Outport  Port=2
  wires:
  Demux/1 -> " Calculate Position and Speed"/1(QEP_Position_Count)
  IndexOffset/1 -> " Calculate Position and Speed"/3(Offset)
  Demux/2 -> " Calculate Position and Speed"/2(QEP_Index_Latch)
  " Calculate Position and Speed"/2(speed) -> speed/1
  " Calculate Position and Speed"/1(Theta_e) -> Theta_e/1
  Qep_Meas/1 -> Demux/1

== system mcb_bldc_sixstep_f28069mLaunchPad_r2020a/Current Control/Inverter/ Code Generation ==
  note: for BoostXL-DRV8305 connected with LaunchXL-28379D
  note: System Outputs
  Inverter Signals : Inport
  Demux1 : Demux  Outputs=6
  Digital Output : c2806xlib/Digital Output  GPIO_Number=GPIO50~GPIO55  GPIO_Bit0=off  GPIO_BIT0_Toggle=off  GPIO_Bit1=off  GPIO_BIT1_Toggle=off  GPIO_Bit2=on  GPIO_BIT2_Toggle=off  GPIO_Bit3=off  GPIO_BIT3_Toggle=off  GPIO_Bit4=off  GPIO_BIT4_Toggle=off  GPIO_Bit5=off  GPIO_BIT5_Toggle=off  GPIO_Bit6=off  GPIO_BIT6_Toggle=off  GPIO_Bit7=off  GPIO_BIT7_Toggle=off
  Enable : DataStoreRead  DataStoreName=Enable
  Ground : Ground
  Mux1 : Mux  Inputs=6
  Scale_to_PWM_Counter_PRD : Gain  Gain=target.PWM_Counter_Period  OutDataTypeStr=uint16  RndMeth=Simplest
  Switch1 : Switch  Threshold=0.5
  ePWM4 : c2802xlib/ePWM  PwmType=C2000  useModule=ePWM1  ePWMxLINKTBPRD=Not Linked  periodUnits=Clock cycles  timerSource=Specify via dialog  timerPeriod_clk=target.PWM_Counter_Period  timerPeriod_sec=64000  tbshadow=Counter equals to zero  countingMode=Up-Down  phaseActiveEnable=Disable  phaseDirection=Count down after sync  phaseActive=0  synchronizationEnable=off  dcaevt1Sync=off  dcbevt1Sync=off  synchronizationOption=Counter equals to zero (CTR=Zero)  dcbevt1SyncOut=off  dcaevt1SyncOut=off  cmpdSyncOut=off  cmpcSyncOut=off  cmpbSyncOut=off  zeroSyncOut=on  swfSyncOut=off  perSynchronizationOption=Counter equals to period (CTR=PRD)  clockPrescale=1  HSclockPrescale=1  enswap=off  ePWMxAStatus=on  ePWMxAactionLogic1=Do nothing  ePWMxAactionLogic2=Do nothing  ePWMxAactionLogic3=Clear  ePWMxAactionLogic4=Set  ePWMxAactionLogic5=Do nothing  ePWMxAactionLogic6=Do nothing  ePWMxACSFenable=off  ePWMxACSFvalue=Forcing disable  ePWMxASFreload=Zero  ePWMxBStatus=on  ePWMxBactionLogic1=Do nothing  ePWMxBactionLogic2=Do nothing  ePWMxBactionLogic3=Do nothing  ePWMxBactionLogic4=Do nothing  ePWMxBactionLogic5=Clear  ePWMxBactionLogic6=Set  ePWMxBCSFenable=off  ePWMxBCSFvalue=Forcing disable  ePWMxBSFreload=Zero  ePWNxBOutWay=off  ePWMxLINKCMPA=Not Linked  CMPAUnits=Clock cycles  CMPASource=Input port  CMPAValue_per=32000  CMPAValue_clk=floor(target.PWM_Counter_Period/2+1)  enCMPAshadow=Counter equals to zero (CTR=Zero)  ePWMxLINKCMPB=Not Linked  CMPBUnits=Clock cycles  CMPBSource=Input port  CMPBValue_per=50  CMPBValue_clk=floor(target.PWM_Counter_Period/2+1)  enCMPBshadow=Counter equals to zero (CTR=Zero)  ePWMxLINKCMPC=Not Linked  CMPCUnits=Clock cycles  CMPCSource=Specify via dialog  CMPCValue_per=50  CMPCValue_clk=32000  enCMPCshadow=Counter equals to zero (CTR=Zero)  ePWMxLINKCMPD=Not Linked  CMPDUnits=Clock cycles  CMPDSource=Specify via dialog  CMPDValue_per=50  CMPDValue_clk=32000  enCMPDshadow=Counter equals to zero (CTR=Zero)  enableDBePWMxA=off  enableDBePWMxB=off  enhalfcycle=off  DBpolarity=Active high complementary (AHC)  DBedgeDelay=Positive  DBSource_ePWMxA=ePWMxA  DBSource_ePWMxB=ePWMxA  DBPeriodUnits=Clock cycles  DBperiodSource=Specify via dialog  REDperiod=15  FEDperiod=15  REDperiod_sec=0  FEDperiod_sec=0  LoadModeDBRED=Immediate without using shadow  LoadModeDBFED=Immediate without using shadow  adcstartModuleA=on  adcrequestEventA=First event  adcstartEventA=Counter equals to zero (CTR=Zero)  adcstartEventA_type2=Digital Compare Module A Event 1 start of conversion (DCAEVT1.soc)  adcstartModuleB=off  adcrequestEventB=First event  adcstartEventB=Counter equals to zero (CTR=Zero)  adcstartEventB_type2=Counter equals to zero (CTR=Zero)  intEn=off  intPrd=First event  intSel=Counter equals to zero (CTR=Zero)  intSel_type2=Counter equals to zero (CTR=Zero)  hrpe=off  enHRPWM=off  HRPWM_LoadMode=Counter equals to period (CTR=PRD)  HRPWM_CTLMode=Duty or Period control mode  HRPWM_EDGMode=Both edge  hrpeb=off  enHRPWMB=off  HRPWM_LoadModeB=Counter equals to zero (CTR=ZERO)  HRPWM_CTLModeB=Duty or Period control mode  HRPWM_EDGModeB=Both edge  enHRDBRED=off  enHRDBFED=off  enSFO=on  enautoconv=on  chopperEnable=off  chopperFrequency=1  chopperFirstwidth=1  chopperDuty=12.5%  tripZonesource=Specify via dialog  tzselOSHT1=off  tzselOSHT2=off  tzselOSHT3=off  tzselOSHDCAEV1=off  tzselOSHDCBEV1=off  tzselCBC1=off  tzselCBC2=off  tzselCBC3=off  tzselCBCDCAEV2=off  tzselCBCDCBEV2=off  tzselOSHT4=off  tzselOSHT5=off  tzselOSHT6=off  tzselCBC4=off  tzselCBC5=off  tzselCBC6=off  enTzOstIntr=off  enTzCbcIntr=off  enTzDCAEVT1Intr=off  enTzDCAEVT2Intr=off  enTzDCBEVT1Intr=off  enTzDCBEVT2Intr=off  ePWMxAforced=No action  ePWMxBforced=No action  DCAEVT1forced=No action  DCBEVT1forced=No action  DCAEVT2forced=No action  DCBEVT2forced=No action  dcah=Trip Zone 1 input (TZ1)  dcal=Trip Zone 2 input (TZ2)  dcbh=Trip Zone 1 input (TZ1)  dcbl=Trip Zone 2 input (TZ2)  dcah_type2=GPTRIP1SEL/(TZ1)  dcal_type2=GPTRIP2SEL/(TZ2)  dcbh_type2=GPTRIP1SEL/(TZ1)  dcbl_type2=GPTRIP2SEL/(TZ2)  gendcaevt1=Event disabled  gendcaevt2=Event disabled  gendcbevt1=Event disabled  gendcbevt2=Event disabled  dcaevt1src=DCAEVT1 with sync  dcaevt2src=DCAEVT2 with sync  dcbevt1src=DCBEVT1 with sync  dcbevt2src=DCBEVT2 with sync  pulsesel=Counter equals to zero (CTR=Zero)  blankinv=off  blankoffset=0  blankwidth=0  evsrcsel=Filtered version of DCAEVT1 (DCAEVT1FILT)  encape=off
  ePWM5 : c2802xlib/ePWM  PwmType=C2000  useModule=ePWM2  ePWMxLINKTBPRD=Not Linked  periodUnits=Clock cycles  timerSource=Specify via dialog  timerPeriod_clk=target.PWM_Counter_Period  timerPeriod_sec=64000  tbshadow=Counter equals to zero  countingMode=Up-Down  phaseActiveEnable=Set counter to phase value specified via dialog  phaseDirection=Count up after sync  phaseActive=0  synchronizationEnable=off  dcaevt1Sync=off  dcbevt1Sync=off  synchronizationOption=Pass through (EPWMxSYNCI or SWFSYNC)  dcbevt1SyncOut=off  dcaevt1SyncOut=off  cmpdSyncOut=off  cmpcSyncOut=off  cmpbSyncOut=off  zeroSyncOut=off  swfSyncOut=on  perSynchronizationOption=Counter equals to period (CTR=PRD)  clockPrescale=1  HSclockPrescale=1  enswap=off  ePWMxAStatus=on  ePWMxAactionLogic1=Do nothing  ePWMxAactionLogic2=Do nothing  ePWMxAactionLogic3=Clear  ePWMxAactionLogic4=Set  ePWMxAactionLogic5=Do nothing  ePWMxAactionLogic6=Do nothing  ePWMxACSFenable=off  ePWMxACSFvalue=Forcing disable  ePWMxASFreload=Zero  ePWMxBStatus=on  ePWMxBactionLogic1=Do nothing  ePWMxBactionLogic2=Do nothing  ePWMxBactionLogic3=Do nothing  ePWMxBactionLogic4=Do nothing  ePWMxBactionLogic5=Clear  ePWMxBactionLogic6=Set  ePWMxBCSFenable=off  ePWMxBCSFvalue=Forcing disable  ePWMxBSFreload=Zero  ePWNxBOutWay=off  ePWMxLINKCMPA=Not Linked  CMPAUnits=Clock cycles  CMPASource=Input port  CMPAValue_per=32000  CMPAValue_clk=floor(target.PWM_Counter_Period/2+1)  enCMPAshadow=Counter equals to zero (CTR=Zero)  ePWMxLINKCMPB=Not Linked  CMPBUnits=Clock cycles  CMPBSource=Input port  CMPBValue_per=50  CMPBValue_clk=floor(target.PWM_Counter_Period/2+1)  enCMPBshadow=Counter equals to zero (CTR=Zero)  ePWMxLINKCMPC=Not Linked  CMPCUnits=Clock cycles  CMPCSource=Specify via dialog  CMPCValue_per=50  CMPCValue_clk=32000  enCMPCshadow=Counter equals to zero (CTR=Zero)  ePWMxLINKCMPD=Not Linked  CMPDUnits=Clock cycles  CMPDSource=Specify via dialog  CMPDValue_per=50  CMPDValue_clk=32000  enCMPDshadow=Counter equals to zero (CTR=Zero)  enableDBePWMxA=off  enableDBePWMxB=off  enhalfcycle=off  DBpolarity=Active high complementary (AHC)  DBedgeDelay=Positive  DBSource_ePWMxA=ePWMxA  DBSource_ePWMxB=ePWMxA  DBPeriodUnits=Clock cycles  DBperiodSource=Specify via dialog  REDperiod=15  FEDperiod=15  REDperiod_sec=0  FEDperiod_sec=0  LoadModeDBRED=Immediate without using shadow  LoadModeDBFED=Immediate without using shadow  adcstartModuleA=off  adcrequestEventA=First event  adcstartEventA=Digital Compare Module A Event 1 start of conversion (DCAEVT1.soc)  adcstartEventA_type2=Digital Compare Module A Event 1 start of conversion (DCAEVT1.soc)  adcstartModuleB=off  adcrequestEventB=First event  adcstartEventB=Counter equals to zero (CTR=Zero)  adcstartEventB_type2=Counter equals to zero (CTR=Zero)  intEn=off  intPrd=First event  intSel=Counter equals to zero (CTR=Zero)  intSel_type2=Counter equals to zero (CTR=Zero)  hrpe=off  enHRPWM=off  HRPWM_LoadMode=Counter equals to period (CTR=PRD)  HRPWM_CTLMode=Duty or Period control mode  HRPWM_EDGMode=Both edge  hrpeb=off  enHRPWMB=off  HRPWM_LoadModeB=Counter equals to zero (CTR=ZERO)  HRPWM_CTLModeB=Duty or Period control mode  HRPWM_EDGModeB=Both edge  enHRDBRED=off  enHRDBFED=off  enSFO=on  enautoconv=on  chopperEnable=off  chopperFrequency=1  chopperFirstwidth=1  chopperDuty=12.5%  tripZonesource=Specify via dialog  tzselOSHT1=off  tzselOSHT2=off  tzselOSHT3=off  tzselOSHDCAEV1=off  tzselOSHDCBEV1=off  tzselCBC1=off  tzselCBC2=off  tzselCBC3=off  tzselCBCDCAEV2=off  tzselCBCDCBEV2=off  tzselOSHT4=off  tzselOSHT5=off  tzselOSHT6=off  tzselCBC4=off  tzselCBC5=off  tzselCBC6=off  enTzOstIntr=off  enTzCbcIntr=off  enTzDCAEVT1Intr=off  enTzDCAEVT2Intr=off  enTzDCBEVT1Intr=off  enTzDCBEVT2Intr=off  ePWMxAforced=No action  ePWMxBforced=No action  DCAEVT1forced=No action  DCBEVT1forced=No action  DCAEVT2forced=No action  DCBEVT2forced=No action  dcah=Trip Zone 1 input (TZ1)  dcal=Trip Zone 2 input (TZ2)  dcbh=Trip Zone 1 input (TZ1)  dcbl=Trip Zone 2 input (TZ2)  dcah_type2=GPTRIP1SEL/(TZ1)  dcal_type2=GPTRIP2SEL/(TZ2)  dcbh_type2=GPTRIP1SEL/(TZ1)  dcbl_type2=GPTRIP2SEL/(TZ2)  gendcaevt1=Event disabled  gendcaevt2=Event disabled  gendcbevt1=Event disabled  gendcbevt2=Event disabled  dcaevt1src=DCAEVT1 with sync  dcaevt2src=DCAEVT2 with sync  dcbevt1src=DCBEVT1 with sync  dcbevt2src=DCBEVT2 with sync  pulsesel=Counter equals to zero (CTR=Zero)  blankinv=off  blankoffset=0  blankwidth=0  evsrcsel=Filtered version of DCAEVT1 (DCAEVT1FILT)  encape=off
  ePWM6 : c2802xlib/ePWM  PwmType=C2000  useModule=ePWM3  ePWMxLINKTBPRD=Not Linked  periodUnits=Clock cycles  timerSource=Specify via dialog  timerPeriod_clk=target.PWM_Counter_Period  timerPeriod_sec=64000  tbshadow=Counter equals to zero  countingMode=Up-Down  phaseActiveEnable=Set counter to phase value specified via dialog  phaseDirection=Count up after sync  phaseActive=0  synchronizationEnable=off  dcaevt1Sync=off  dcbevt1Sync=off  synchronizationOption=Disable  dcbevt1SyncOut=off  dcaevt1SyncOut=off  cmpdSyncOut=off  cmpcSyncOut=off  cmpbSyncOut=off  zeroSyncOut=off  swfSyncOut=off  perSynchronizationOption=Counter equals to period (CTR=PRD)  clockPrescale=1  HSclockPrescale=1  enswap=off  ePWMxAStatus=on  ePWMxAactionLogic1=Do nothing  ePWMxAactionLogic2=Do nothing  ePWMxAactionLogic3=Clear  ePWMxAactionLogic4=Set  ePWMxAactionLogic5=Do nothing  ePWMxAactionLogic6=Do nothing  ePWMxACSFenable=off  ePWMxACSFvalue=Forcing disable  ePWMxASFreload=Zero  ePWMxBStatus=on  ePWMxBactionLogic1=Do nothing  ePWMxBactionLogic2=Do nothing  ePWMxBactionLogic3=Do nothing  ePWMxBactionLogic4=Do nothing  ePWMxBactionLogic5=Clear  ePWMxBactionLogic6=Set  ePWMxBCSFenable=off  ePWMxBCSFvalue=Forcing disable  ePWMxBSFreload=Zero  ePWNxBOutWay=off  ePWMxLINKCMPA=Not Linked  CMPAUnits=Clock cycles  CMPASource=Input port  CMPAValue_per=32000  CMPAValue_clk=floor(target.PWM_Counter_Period/2+1)  enCMPAshadow=Counter equals to zero (CTR=Zero)  ePWMxLINKCMPB=Not Linked  CMPBUnits=Clock cycles  CMPBSource=Input port  CMPBValue_per=50  CMPBValue_clk=floor(target.PWM_Counter_Period/2+1)  enCMPBshadow=Counter equals to zero (CTR=Zero)  ePWMxLINKCMPC=Not Linked  CMPCUnits=Clock cycles  CMPCSource=Specify via dialog  CMPCValue_per=50  CMPCValue_clk=32000  enCMPCshadow=Counter equals to zero (CTR=Zero)  ePWMxLINKCMPD=Not Linked  CMPDUnits=Clock cycles  CMPDSource=Specify via dialog  CMPDValue_per=50  CMPDValue_clk=32000  enCMPDshadow=Counter equals to zero (CTR=Zero)  enableDBePWMxA=off  enableDBePWMxB=off  enhalfcycle=off  DBpolarity=Active high complementary (AHC)  DBedgeDelay=Positive  DBSource_ePWMxA=ePWMxA  DBSource_ePWMxB=ePWMxA  DBPeriodUnits=Clock cycles  DBperiodSource=Specify via dialog  REDperiod=15  FEDperiod=15  REDperiod_sec=0  FEDperiod_sec=0  LoadModeDBRED=Immediate without using shadow  LoadModeDBFED=Immediate without using shadow  adcstartModuleA=off  adcrequestEventA=First event  adcstartEventA=Digital Compare Module A Event 1 start of conversion (DCAEVT1.soc)  adcstartEventA_type2=Digital Compare Module A Event 1 start of conversion (DCAEVT1.soc)  adcstartModuleB=off  adcrequestEventB=First event  adcstartEventB=Counter equals to zero (CTR=Zero)  adcstartEventB_type2=Counter equals to zero (CTR=Zero)  intEn=off  intPrd=First event  intSel=Counter equals to zero (CTR=Zero)  intSel_type2=Counter equals to zero (CTR=Zero)  hrpe=off  enHRPWM=off  HRPWM_LoadMode=Counter equals to period (CTR=PRD)  HRPWM_CTLMode=Duty or Period control mode  HRPWM_EDGMode=Both edge  hrpeb=off  enHRPWMB=off  HRPWM_LoadModeB=Counter equals to zero (CTR=ZERO)  HRPWM_CTLModeB=Duty or Period control mode  HRPWM_EDGModeB=Both edge  enHRDBRED=off  enHRDBFED=off  enSFO=on  enautoconv=on  chopperEnable=off  chopperFrequency=1  chopperFirstwidth=1  chopperDuty=12.5%  tripZonesource=Specify via dialog  tzselOSHT1=off  tzselOSHT2=off  tzselOSHT3=off  tzselOSHDCAEV1=off  tzselOSHDCBEV1=off  tzselCBC1=off  tzselCBC2=off  tzselCBC3=off  tzselCBCDCAEV2=off  tzselCBCDCBEV2=off  tzselOSHT4=off  tzselOSHT5=off  tzselOSHT6=off  tzselCBC4=off  tzselCBC5=off  tzselCBC6=off  enTzOstIntr=off  enTzCbcIntr=off  enTzDCAEVT1Intr=off  enTzDCAEVT2Intr=off  enTzDCBEVT1Intr=off  enTzDCBEVT2Intr=off  ePWMxAforced=No action  ePWMxBforced=No action  DCAEVT1forced=No action  DCBEVT1forced=No action  DCAEVT2forced=No action  DCBEVT2forced=No action  dcah=Trip Zone 1 input (TZ1)  dcal=Trip Zone 2 input (TZ2)  dcbh=Trip Zone 1 input (TZ1)  dcbl=Trip Zone 2 input (TZ2)  dcah_type2=GPTRIP1SEL/(TZ1)  dcal_type2=GPTRIP2SEL/(TZ2)  dcbh_type2=GPTRIP1SEL/(TZ1)  dcbl_type2=GPTRIP2SEL/(TZ2)  gendcaevt1=Event disabled  gendcaevt2=Event disabled  gendcbevt1=Event disabled  gendcbevt2=Event disabled  dcaevt1src=DCAEVT1 with sync  dcaevt2src=DCAEVT2 with sync  dcbevt1src=DCBEVT1 with sync  dcbevt2src=DCBEVT2 with sync  pulsesel=Counter equals to zero (CTR=Zero)  blankinv=off  blankoffset=0  blankwidth=0  evsrcsel=Filtered version of DCAEVT1 (DCAEVT1FILT)  encape=off
  stop : Constant  Value=[0 0 0 0 0 0]  OutDataTypeStr=uint16
  Duty : Outport  VectorParamsAs1DForOutWhenUnconnected=off
  wires:
  Scale_to_PWM_Counter_PRD/1 -> Switch1/1
  stop/1 -> Switch1/3
  Switch1/1 -> Demux1/1
  Ground/1 -> Mux1/6, Mux1/5, Mux1/4, Mux1/3, Mux1/2, Mux1/1
  Mux1/1 -> Duty/1
  Inverter Signals/1 -> Scale_to_PWM_Counter_PRD/1  "PWM Duty Cycles"
  Enable/1 -> Digital Output/1, Switch1/2
  Demux1/1 -> ePWM4/1  "PWM_A"
  Demux1/2 -> ePWM4/2  "PWM_B"
  Demux1/3 -> ePWM5/1  "PWM_C"
  Demux1/4 -> ePWM5/2
  Demux1/5 -> ePWM6/1
  Demux1/6 -> ePWM6/2

== system mcb_bldc_sixstep_f28069mLaunchPad_r2020a/Current Control/Inverter/Simulation ==
  Inverter Signals : Inport
  Data Type Duplicate : DataTypeDuplicate
  Enable : DataStoreRead  DataStoreName=Enable
  Switch1 : Switch  Threshold=0.5  RndMeth=Simplest
  stop : Constant  Value=[0 0 0 0 0 0]  OutDataTypeStr=Inherit: Inherit via back propagation
  Duty : Outport  VectorParamsAs1DForOutWhenUnconnected=off
  wires:
  stop/1 -> Switch1/3, Data Type Duplicate/2
  Switch1/1 -> Duty/1
  Inverter Signals/1 -> Data Type Duplicate/1, Switch1/1  "PWM Duty Cycles"
  Enable/1 -> Switch1/2

== system mcb_bldc_sixstep_f28069mLaunchPad_r2020a/Current Control/SCI_Tx/ Code Generation ==
  SCI_Data : Inport
  CodeGeneration : Subsystem  TreatAsAtomicUnit=on
  wires:
  SCI_Data/1 -> CodeGeneration/1(Input)

== system mcb_bldc_sixstep_f28069mLaunchPad_r2020a/Current Control/SCI_Tx/Simulation ==
  SCI_Data : Inport
  Demux : Demux  Outputs=2
  Terminator1 : Terminator
  Terminator2 : Terminator
  wires:
  SCI_Data/1 -> Demux/1
  Demux/1 -> Terminator1/1
  Demux/2 -> Terminator2/1
